simulink model "sampleModel7293_pp_1_1_mu"  (R2018a)
settings: Solver=VariableStepAuto  StartTime=0.0  StopTime=10.0  RelTol=1e-3
undefined symbols (not defined in the file): DiscIntNeverNeededParam
libraries: simulink x367
(part 9 of 13)

== system sampleModel7293_pp_1_1_mu/cfblk193/emi_96 ==
  Action Port : ActionPort  ActionType=else
  emi_97 : Assertion

== system sampleModel7293_pp_1_1_mu/cfblk194/cfblk4 ==
  emi_516 : Inport
  Action Port : ActionPort  ActionType=then
  cfblk4 : simulink/Continuous/PID Controller  Controller=PID  TimeDomain=Discrete-time  SampleTime=-1  IntegratorMethod=Forward Euler  FilterMethod=Forward Euler  Form=Parallel  UseFilter=on  ControllerParametersSource=internal  P=1  I=1  D=0  N=100  InitialConditionSource=internal  InitialConditionForIntegrator=0  InitialConditionForFilter=0  ExternalReset=none  LimitOutput=off  UpperSaturationLimit=inf  LowerSaturationLimit=-inf  LinearizeAsGain=off  AntiWindupMode=none  Kb=1  TrackingMode=off  Kt=1  PParamMin=[]  PParamMax=[]  IParamMin=[]  IParamMax=[]  DParamMin=[]  DParamMax=[]  NParamMin=[]  NParamMax=[]  KbParamMin=[]  KbParamMax=[]  KtParamMin=[]  KtParamMax=[]  POutMin=[]  POutMax=[]  IOutMin=[]  IOutMax=[]  DOutMin=[]  DOutMax=[]  NOutMin=[]  NOutMax=[]  KbOutMin=[]  KbOutMax=[]  KtOutMin=[]  KtOutMax=[]  IntegratorOutMin=[]  IntegratorOutMax=[]  FilterOutMin=[]  FilterOutMax=[]  SumOutMin=[]  SumOutMax=[]  SumI1OutMin=[]  SumI1OutMax=[]  SumI2OutMin=[]  SumI2OutMax=[]  SumI3OutMin=[]  SumI3OutMax=[]  SumDOutMin=[]  SumDOutMax=[]  SaturationOutMin=[]  SaturationOutMax=[]  IntegratorContinuousStateAttributes=''  IntegratorStateMustResolveToSignalObject=off  IntegratorRTWStateStorageClass=Auto  FilterContinuousStateAttributes=''  FilterStateMustResolveToSignalObject=off  FilterRTWStateStorageClass=Auto  DifferentiatorICPrevScaledInput=0  DifferentiatorOutMin=[]  DifferentiatorOutMax=[]  FilterDiffOutCoefMin=[]  FilterDiffOutCoefMax=[]  SumDenOutMin=[]  SumDenOutMax=[]  SumNumOutMin=[]  SumNumOutMax=[]  ReciprocalOutMin=[]  ReciprocalOutMax=[]  DivideOutMin=[]  DivideOutMax=[]  TunerSelectOption=Transfer Function Based (PID Tuner App)
  emi_517 : Outport
  wires:
  emi_516/1 -> cfblk4/1
  cfblk4/1 -> emi_517/1

== system sampleModel7293_pp_1_1_mu/cfblk194/cfblk5 ==
  emi_509 : Inport
  Action Port : ActionPort  ActionType=then
  cfblk5 : UnitDelay  SampleTime=-1
  emi_510 : Outport
  wires:
  emi_509/1 -> cfblk5/1
  cfblk5/1 -> emi_510/1

== system sampleModel7293_pp_1_1_mu/cfblk194/cfblk6 ==
  emi_208 : Inport
  Action Port : ActionPort  ActionType=then
  cfblk6 : DiscreteTransferFcn
  emi_209 : Outport
  wires:
  emi_208/1 -> cfblk6/1
  cfblk6/1 -> emi_209/1

== system sampleModel7293_pp_1_1_mu/cfblk194/cfblk7 ==
  emi_64 : Inport
  emi_65 : Inport  Port=2
  Action Port : ActionPort  ActionType=then
  cfblk7 : Delay  ShowEnablePort=on
      settings: InputPortMap=u0,e6
  emi_66 : Outport
  wires:
  emi_64/1 -> cfblk7/1
  emi_65/1 -> cfblk7/2
  cfblk7/1 -> emi_66/1

== system sampleModel7293_pp_1_1_mu/cfblk194/cfblk8 ==
  emi_1728 : Inport
  Action Port : ActionPort  ActionType=then
  cfblk8 : Delay
  emi_1729 : Outport
  wires:
  emi_1728/1 -> cfblk8/1
  cfblk8/1 -> emi_1729/1

== system sampleModel7293_pp_1_1_mu/cfblk194/emi_1730 ==
  Action Port : ActionPort  ActionType=else
  emi_1731 : Assertion

== system sampleModel7293_pp_1_1_mu/cfblk194/emi_210 ==
  Action Port : ActionPort  ActionType=else
  emi_211 : Assertion

== system sampleModel7293_pp_1_1_mu/cfblk194/emi_511 ==
  Action Port : ActionPort  ActionType=else
  emi_512 : Assertion

== system sampleModel7293_pp_1_1_mu/cfblk194/emi_518 ==
  Action Port : ActionPort  ActionType=else
  emi_519 : Assertion

== system sampleModel7293_pp_1_1_mu/cfblk194/emi_67 ==
  Action Port : ActionPort  ActionType=else
  emi_68 : Assertion

== system sampleModel7293_pp_1_1_mu/cfblk195/cfblk11 ==
  emi_157 : Inport
  Action Port : ActionPort  ActionType=then
  cfblk11 : Delay
  emi_158 : Outport
  wires:
  emi_157/1 -> cfblk11/1
  cfblk11/1 -> emi_158/1

== system sampleModel7293_pp_1_1_mu/cfblk195/cfblk4 ==
  emi_387 : Inport
  Action Port : ActionPort  ActionType=then
  cfblk4 : simulink/Discrete/Difference  ICPrevInput=0.0  OutMin=[]  OutMax=[]  OutDataTypeStr=double  OutputDataTypeScalingMode=double  OutDataType=fixdt(1, 16)  OutScaling=2^-10  DoSatur=off
  emi_388 : Outport
  wires:
  emi_387/1 -> cfblk4/1
  cfblk4/1 -> emi_388/1

== system sampleModel7293_pp_1_1_mu/cfblk195/cfblk8 ==
  cfblk1 : Inport
  cfblk11 : Inport  Port=2
  cfblk12 : Inport  Port=3
  Action Port : ActionPort  ActionType=then
  cfblk10 : simulink/Continuous/PID Controller (2DOF)  Controller=PID  TimeDomain=Discrete-time  SampleTime=-1  IntegratorMethod=Forward Euler  FilterMethod=Forward Euler  Form=Parallel  UseFilter=on  ControllerParametersSource=internal  P=1  I=1  D=0  N=100  b=1  c=1  InitialConditionSource=internal  InitialConditionForIntegrator=0  InitialConditionForFilter=0  ExternalReset=none  LimitOutput=off  UpperSaturationLimit=inf  LowerSaturationLimit=-inf  LinearizeAsGain=off  AntiWindupMode=none  Kb=1  TrackingMode=off  Kt=1  PParamMin=[]  PParamMax=[]  IParamMin=[]  IParamMax=[]  DParamMin=[]  DParamMax=[]  NParamMin=[]  NParamMax=[]  bParamMin=[]  bParamMax=[]  cParamMin=[]  cParamMax=[]  KbParamMin=[]  KbParamMax=[]  KtParamMin=[]  KtParamMax=[]  POutMin=[]  POutMax=[]  IOutMin=[]  IOutMax=[]  DOutMin=[]  DOutMax=[]  NOutMin=[]  NOutMax=[]  bOutMin=[]  bOutMax=[]  cOutMin=[]  cOutMax=[]  KbOutMin=[]  KbOutMax=[]  KtOutMin=[]  KtOutMax=[]  IntegratorOutMin=[]  IntegratorOutMax=[]  FilterOutMin=[]  FilterOutMax=[]  SumOutMin=[]  SumOutMax=[]  Sum1OutMin=[]  Sum1OutMax=[]  Sum2OutMin=[]  Sum2OutMax=[]  Sum3OutMin=[]  Sum3OutMax=[]  SumI1OutMin=[]  SumI1OutMax=[]  SumI2OutMin=[]  SumI2OutMax=[]  SumI3OutMin=[]  SumI3OutMax=[]  SumDOutMin=[]  SumDOutMax=[]  SaturationOutMin=[]  SaturationOutMax=[]  IntegratorContinuousStateAttributes=''  IntegratorStateMustResolveToSignalObject=off  IntegratorRTWStateStorageClass=Auto  FilterContinuousStateAttributes=''  FilterStateMustResolveToSignalObject=off  FilterRTWStateStorageClass=Auto  DifferentiatorICPrevScaledInput=0  DifferentiatorOutMin=[]  DifferentiatorOutMax=[]  FilterDiffOutCoefMin=[]  FilterDiffOutCoefMax=[]  SumDenOutMin=[]  SumDenOutMax=[]  SumNumOutMin=[]  SumNumOutMax=[]  ReciprocalOutMin=[]  ReciprocalOutMax=[]  DivideOutMin=[]  DivideOutMax=[]  TunerSelectOption=Transfer Function Based (PID Tuner App)
  cfblk13 : Subsystem  TreatAsAtomicUnit=on
  cfblk3 : simulink/Discrete/Transfer Fcn Real Zero  ZeroZ=0.75  ICPrevInput=0.0  DoSatur=off
      settings: SourceProductName=Simulink  SourceProductBaseCode=SL
  cfblk4 : Delay  ShowEnablePort=on
      settings: InputPortMap=u0,e6
  cfblk5 : simulink/Discrete/Transfer Fcn First Order  PoleZ=0.95  ICPrevOutput=0.0  DoSatur=off
      settings: SourceProductName=Simulink
  cfblk6 : UnitDelay  SampleTime=-1
  cfblk7 : UnitDelay  SampleTime=-1
  cfblk8 : Subsystem  TreatAsAtomicUnit=on
  cfblk9 : Subsystem  TreatAsAtomicUnit=on
  cyemi_{892..902} (11 alike) : DataTypeConversion  OutDataTypeStr=double
  emi_1595 : Subsystem  TreatAsAtomicUnit=on
  emi_1597 : If  IfExpression=Inf <= u1
  emi_1598 : DataTypeConversion  OutDataTypeStr=double
  emi_1993 : Subsystem  TreatAsAtomicUnit=on
  emi_1995 : If  IfExpression=Inf <= u1
  emi_1996 : DataTypeConversion  OutDataTypeStr=double
  emi_497 : Subsystem  TreatAsAtomicUnit=on
  emi_499 : If  IfExpression=Inf <= u1
  emi_500 : DataTypeConversion  OutDataTypeStr=double
  cfblk2 : Outport
  wires:
  cfblk4/1 -> cyemi_898/1, cyemi_899/1
  cfblk10/1 -> cfblk2/1
  cyemi_892/1 -> cfblk10/1
  cfblk7/1 -> cyemi_892/1, emi_1598/1, emi_1996/1
  cyemi_893/1 -> cfblk10/2
  cfblk3/1 -> cyemi_893/1
  cyemi_895/1 -> cfblk3/1
  cfblk1/1 -> cyemi_895/1
  cyemi_896/1 -> cfblk4/1
  cfblk11/1 -> cyemi_896/1
  cyemi_897/1 -> cfblk4/2
  cyemi_898/1 -> cfblk5/1
  cyemi_899/1 -> cfblk6/1
  cyemi_900/1 -> cfblk7/1
  cfblk12/1 -> cyemi_900/1
  cfblk6/1 -> cyemi_902/1
  cyemi_901/1 -> cfblk8/1(emi_495)
  cfblk8/1(emi_496) -> cyemi_894/1
  emi_499/1 -> cfblk8/Action
  emi_499/2 -> emi_497/Action
  emi_500/1 -> emi_499/1
  cyemi_894/1 -> cfblk13/1(emi_1593)
  cfblk13/1(emi_1594) -> emi_500/1, cyemi_897/1
  emi_1597/1 -> cfblk13/Action
  emi_1597/2 -> emi_1595/Action
  emi_1598/1 -> emi_1597/1
  cyemi_902/1 -> cfblk9/1(emi_1991)
  cfblk9/1(emi_1992) -> cyemi_901/1
  emi_1995/1 -> cfblk9/Action
  emi_1995/2 -> emi_1993/Action
  emi_1996/1 -> emi_1995/1

== system sampleModel7293_pp_1_1_mu/cfblk195/cfblk9 ==
  cfblk1 : Inport
  cfblk11 : Inport  Port=2
  cfblk12 : Inport  Port=3
  cfblk13 : Inport  Port=4
  Action Port : ActionPort  ActionType=else
  cfblk10 : DiscreteZeroPole  Poles=[0 0.5]  Gain=1  SampleTime=-1
  cfblk3 : simulink/Discrete/Transfer Fcn Real Zero  ZeroZ=0.75  ICPrevInput=0.0  DoSatur=off
      settings: SourceProductName=Simulink  SourceProductBaseCode=SL
  cfblk4 : DiscreteFir
  cfblk5 : DiscreteFilter
  cfblk6 : Delay  ShowEnablePort=on
      settings: InputPortMap=u0,e6
  cfblk7 : DiscreteIntegrator  SampleTime=-1  OutDataTypeStr=double  ICPrevOutput=DiscIntNeverNeededParam  ICPrevScaledInput=DiscIntNeverNeededParam
  cfblk8 : UnitDelay  SampleTime=-1
  cfblk9 : Subsystem  TreatAsAtomicUnit=on
  cyemi_{907..915} (9 alike) : DataTypeConversion  OutDataTypeStr=double
  emi_1588 : Subsystem  TreatAsAtomicUnit=on
  emi_1590 : If  IfExpression=0 <= u1
  emi_1591 : DataTypeConversion  OutDataTypeStr=double
  cfblk2 : Outport
  cfblk14 : Outport  Port=2
  cfblk15 : Outport  Port=3
  wires:
  cfblk12/1 -> cfblk2/1
  cfblk6/1 -> cfblk14/1
  cyemi_907/1 -> cfblk10/1
  cfblk13/1 -> cyemi_907/1
  cyemi_908/1 -> cfblk3/1
  cfblk11/1 -> cyemi_908/1
  cyemi_909/1 -> cfblk4/1
  cfblk8/1 -> cyemi_909/1
  cyemi_910/1 -> cfblk5/1
  cfblk4/1 -> cyemi_910/1, emi_1591/1
  cyemi_911/1 -> cfblk6/1
  cfblk5/1 -> cyemi_911/1
  cyemi_912/1 -> cfblk6/2
  cfblk7/1 -> cyemi_912/1
  cyemi_913/1 -> cfblk7/1
  cfblk10/1 -> cyemi_913/1
  cyemi_914/1 -> cfblk8/1
  cfblk3/1 -> cyemi_914/1
  cfblk1/1 -> cyemi_915/1
  cyemi_915/1 -> cfblk9/1(emi_1586)
  cfblk9/1(emi_1587) -> cfblk15/1
  emi_1590/1 -> cfblk9/Action
  emi_1590/2 -> emi_1588/Action
  emi_1591/1 -> emi_1590/1

== system sampleModel7293_pp_1_1_mu/cfblk195/emi_159 ==
  Action Port : ActionPort  ActionType=else
  emi_160 : Assertion

== system sampleModel7293_pp_1_1_mu/cfblk195/emi_389 ==
  Action Port : ActionPort  ActionType=else
  emi_390 : Assertion

== system sampleModel7293_pp_1_1_mu/cfblk196/cfblk11 ==
  cfblk1 : Inport
  cfblk10 : Inport  Port=2
  cfblk11 : Inport  Port=3
  Action Port : ActionPort  ActionType=then
  cfblk3 : Subsystem  TreatAsAtomicUnit=on
  cfblk4 : DiscreteStateSpace  SampleTime=-1
  cfblk5 : simulink/Discrete/Transfer Fcn First Order  PoleZ=0.95  ICPrevOutput=0.0  DoSatur=off
      settings: SourceProductName=Simulink
  cfblk6 : simulink/Discrete/Transfer Fcn First Order  PoleZ=0.95  ICPrevOutput=0.0  DoSatur=off
      settings: SourceProductName=Simulink
  cfblk7 : DiscreteFilter
  cfblk8 : simulink/Discrete/Transfer Fcn Lead or Lag  PoleZ=0.95  ZeroZ=0.75  ICPrevOutput=0.0  ICPrevInput=0.0  DoSatur=off
      settings: SourceProductName=Simulink  SourceProductBaseCode=SL
  cfblk9 : simulink/Discrete/Tapped Delay  vinit=0.0  samptime=-1  NumDelays=1  DelayOrder=Oldest  includeCurrent=off
  cyemi_{922..928} (7 alike) : DataTypeConversion  OutDataTypeStr=double
  emi_1152 : Subsystem  TreatAsAtomicUnit=on
  emi_1154 : If  IfExpression=Inf <= u1
  emi_1155 : DataTypeConversion  OutDataTypeStr=double
  cfblk2 : Outport
  cfblk12 : Outport  Port=2
  cfblk13 : Outport  Port=3
  wires:
  cfblk4/1 -> cfblk13/1, emi_1155/1
  cfblk9/1 -> cfblk2/1
  cfblk1/1 -> cyemi_924/1, cyemi_925/1
  cfblk7/1 -> cyemi_922/1
  cyemi_923/1 -> cfblk4/1
  cfblk6/1 -> cyemi_923/1
  cyemi_924/1 -> cfblk5/1
  cyemi_925/1 -> cfblk6/1
  cyemi_926/1 -> cfblk7/1
  cfblk8/1 -> cyemi_926/1
  cyemi_927/1 -> cfblk8/1
  cfblk11/1 -> cyemi_927/1
  cyemi_928/1 -> cfblk9/1
  cfblk10/1 -> cyemi_928/1
  cyemi_922/1 -> cfblk3/1(emi_1150)
  cfblk3/1(emi_1151) -> cfblk12/1
  emi_1154/1 -> cfblk3/Action
  emi_1154/2 -> emi_1152/Action
  emi_1155/1 -> emi_1154/1

== system sampleModel7293_pp_1_1_mu/cfblk196/cfblk12 ==
  cfblk1 : Inport
  Action Port : ActionPort  ActionType=else
  cfblk10 : DiscreteZeroPole  Poles=[0 0.5]  Gain=1  SampleTime=-1
  cfblk11 : DiscreteIntegrator  SampleTime=-1  OutDataTypeStr=double  ICPrevOutput=DiscIntNeverNeededParam  ICPrevScaledInput=DiscIntNeverNeededParam
  cfblk13 : Delay
  cfblk3 : Subsystem  TreatAsAtomicUnit=on
  cfblk4 : DiscreteFir
  cfblk5 : simulink/Discrete/Transfer Fcn Lead or Lag  PoleZ=0.95  ZeroZ=0.75  ICPrevOutput=0.0  ICPrevInput=0.0  DoSatur=off
      settings: SourceProductName=Simulink  SourceProductBaseCode=SL
  cfblk6 : DiscreteFir
  cfblk7 : simulink/Discrete/Difference  ICPrevInput=0.0  OutMin=[]  OutMax=[]  OutDataTypeStr=double  OutputDataTypeScalingMode=double  OutDataType=fixdt(1, 16)  OutScaling=2^-10  DoSatur=off
  cfblk8 : DiscreteFilter
  cfblk9 : Subsystem  TreatAsAtomicUnit=on
  cyemi_{930..939} (10 alike) : DataTypeConversion  OutDataTypeStr=double
  emi_1823 : Subsystem  TreatAsAtomicUnit=on
  emi_1825 : If  IfExpression=Inf <= u1
  emi_1826 : DataTypeConversion  OutDataTypeStr=double
  emi_569 : Subsystem  TreatAsAtomicUnit=on
  emi_571 : If  IfExpression=Inf <= u1
  emi_572 : DataTypeConversion  OutDataTypeStr=double
  cfblk2 : Outport
  cfblk12 : Outport  Port=2
  wires:
  cfblk10/1 -> cfblk12/1, cfblk2/1
  cyemi_930/1 -> cfblk10/1
  cfblk5/1 -> cyemi_930/1
  cyemi_931/1 -> cfblk11/1
  cfblk8/1 -> cyemi_931/1
  cyemi_932/1 -> cfblk13/1
  cfblk4/1 -> cyemi_933/1, emi_572/1, emi_1826/1
  cyemi_934/1 -> cfblk4/1
  cfblk11/1 -> cyemi_934/1
  cyemi_935/1 -> cfblk5/1
  cyemi_936/1 -> cfblk6/1
  cfblk13/1 -> cyemi_936/1
  cyemi_937/1 -> cfblk7/1
  cfblk1/1 -> cyemi_937/1
  cyemi_938/1 -> cfblk8/1
  cfblk7/1 -> cyemi_938/1
  cfblk6/1 -> cyemi_939/1
  cyemi_939/1 -> cfblk9/1(emi_567)
  cfblk9/1(emi_568) -> cyemi_932/1
  emi_571/1 -> cfblk9/Action
  emi_571/2 -> emi_569/Action
  emi_572/1 -> emi_571/1
  cyemi_933/1 -> cfblk3/1(emi_1821)
  cfblk3/1(emi_1822) -> cyemi_935/1
  emi_1825/1 -> cfblk3/Action
  emi_1825/2 -> emi_1823/Action
  emi_1826/1 -> emi_1825/1

== system sampleModel7293_pp_1_1_mu/cfblk196/cfblk3 ==
  emi_229 : Inport
  Action Port : ActionPort  ActionType=then
  cfblk3 : simulink/Continuous/PID Controller  Controller=PID  TimeDomain=Discrete-time  SampleTime=-1  IntegratorMethod=Forward Euler  FilterMethod=Forward Euler  Form=Parallel  UseFilter=on  ControllerParametersSource=internal  P=1  I=1  D=0  N=100  InitialConditionSource=internal  InitialConditionForIntegrator=0  InitialConditionForFilter=0  ExternalReset=none  LimitOutput=off  UpperSaturationLimit=inf  LowerSaturationLimit=-inf  LinearizeAsGain=off  AntiWindupMode=none  Kb=1  TrackingMode=off  Kt=1  PParamMin=[]  PParamMax=[]  IParamMin=[]  IParamMax=[]  DParamMin=[]  DParamMax=[]  NParamMin=[]  NParamMax=[]  KbParamMin=[]  KbParamMax=[]  KtParamMin=[]  KtParamMax=[]  POutMin=[]  POutMax=[]  IOutMin=[]  IOutMax=[]  DOutMin=[]  DOutMax=[]  NOutMin=[]  NOutMax=[]  KbOutMin=[]  KbOutMax=[]  KtOutMin=[]  KtOutMax=[]  IntegratorOutMin=[]  IntegratorOutMax=[]  FilterOutMin=[]  FilterOutMax=[]  SumOutMin=[]  SumOutMax=[]  SumI1OutMin=[]  SumI1OutMax=[]  SumI2OutMin=[]  SumI2OutMax=[]  SumI3OutMin=[]  SumI3OutMax=[]  SumDOutMin=[]  SumDOutMax=[]  SaturationOutMin=[]  SaturationOutMax=[]  IntegratorContinuousStateAttributes=''  IntegratorStateMustResolveToSignalObject=off  IntegratorRTWStateStorageClass=Auto  FilterContinuousStateAttributes=''  FilterStateMustResolveToSignalObject=off  FilterRTWStateStorageClass=Auto  DifferentiatorICPrevScaledInput=0  DifferentiatorOutMin=[]  DifferentiatorOutMax=[]  FilterDiffOutCoefMin=[]  FilterDiffOutCoefMax=[]  SumDenOutMin=[]  SumDenOutMax=[]  SumNumOutMin=[]  SumNumOutMax=[]  ReciprocalOutMin=[]  ReciprocalOutMax=[]  DivideOutMin=[]  DivideOutMax=[]  TunerSelectOption=Transfer Function Based (PID Tuner App)
  emi_230 : Outport
  wires:
  emi_229/1 -> cfblk3/1
  cfblk3/1 -> emi_230/1

== system sampleModel7293_pp_1_1_mu/cfblk196/cfblk4 ==
  emi_308 : Inport
  Action Port : ActionPort  ActionType=then
  cfblk4 : simulink/Discrete/Transfer Fcn Lead or Lag  PoleZ=0.95  ZeroZ=0.75  ICPrevOutput=0.0  ICPrevInput=0.0  DoSatur=off
      settings: SourceProductName=Simulink  SourceProductBaseCode=SL
  emi_309 : Outport
  wires:
  emi_308/1 -> cfblk4/1
  cfblk4/1 -> emi_309/1

== system sampleModel7293_pp_1_1_mu/cfblk196/cfblk7 ==
  emi_1657 : Inport
  Action Port : ActionPort  ActionType=then
  cfblk7 : DiscreteIntegrator  SampleTime=-1  OutDataTypeStr=double  ICPrevOutput=DiscIntNeverNeededParam  ICPrevScaledInput=DiscIntNeverNeededParam
  emi_1658 : Outport
  wires:
  emi_1657/1 -> cfblk7/1
  cfblk7/1 -> emi_1658/1

== system sampleModel7293_pp_1_1_mu/cfblk196/emi_1659 ==
  Action Port : ActionPort  ActionType=else
  emi_1660 : Assertion

== system sampleModel7293_pp_1_1_mu/cfblk196/emi_231 ==
  Action Port : ActionPort  ActionType=else
  emi_232 : Assertion

== system sampleModel7293_pp_1_1_mu/cfblk196/emi_310 ==
  Action Port : ActionPort  ActionType=else
  emi_311 : Assertion

== system sampleModel7293_pp_1_1_mu/cfblk197/cfblk16 ==
  cfblk1 : Inport
  Action Port : ActionPort  ActionType=then
  cfblk10 : DiscreteIntegrator  SampleTime=-1  OutDataTypeStr=double  ICPrevOutput=DiscIntNeverNeededParam  ICPrevScaledInput=DiscIntNeverNeededParam
  cfblk{8,14..16} (4 alike) : Delay
  cfblk3 : simulink/Discrete/Difference  ICPrevInput=0.0  OutMin=[]  OutMax=[]  OutDataTypeStr=double  OutputDataTypeScalingMode=double  OutDataType=fixdt(1, 16)  OutScaling=2^-10  DoSatur=off
  cfblk4 : Subsystem  TreatAsAtomicUnit=on
  cfblk5 : simulink/Continuous/PID Controller (2DOF)  Controller=PID  TimeDomain=Discrete-time  SampleTime=-1  IntegratorMethod=Forward Euler  FilterMethod=Forward Euler  Form=Parallel  UseFilter=on  ControllerParametersSource=internal  P=1  I=1  D=0  N=100  b=1  c=1  InitialConditionSource=internal  InitialConditionForIntegrator=0  InitialConditionForFilter=0  ExternalReset=none  LimitOutput=off  UpperSaturationLimit=inf  LowerSaturationLimit=-inf  LinearizeAsGain=off  AntiWindupMode=none  Kb=1  TrackingMode=off  Kt=1  PParamMin=[]  PParamMax=[]  IParamMin=[]  IParamMax=[]  DParamMin=[]  DParamMax=[]  NParamMin=[]  NParamMax=[]  bParamMin=[]  bParamMax=[]  cParamMin=[]  cParamMax=[]  KbParamMin=[]  KbParamMax=[]  KtParamMin=[]  KtParamMax=[]  POutMin=[]  POutMax=[]  IOutMin=[]  IOutMax=[]  DOutMin=[]  DOutMax=[]  NOutMin=[]  NOutMax=[]  bOutMin=[]  bOutMax=[]  cOutMin=[]  cOutMax=[]  KbOutMin=[]  KbOutMax=[]  KtOutMin=[]  KtOutMax=[]  IntegratorOutMin=[]  IntegratorOutMax=[]  FilterOutMin=[]  FilterOutMax=[]  SumOutMin=[]  SumOutMax=[]  Sum1OutMin=[]  Sum1OutMax=[]  Sum2OutMin=[]  Sum2OutMax=[]  Sum3OutMin=[]  Sum3OutMax=[]  SumI1OutMin=[]  SumI1OutMax=[]  SumI2OutMin=[]  SumI2OutMax=[]  SumI3OutMin=[]  SumI3OutMax=[]  SumDOutMin=[]  SumDOutMax=[]  SaturationOutMin=[]  SaturationOutMax=[]  IntegratorContinuousStateAttributes=''  IntegratorStateMustResolveToSignalObject=off  IntegratorRTWStateStorageClass=Auto  FilterContinuousStateAttributes=''  FilterStateMustResolveToSignalObject=off  FilterRTWStateStorageClass=Auto  DifferentiatorICPrevScaledInput=0  DifferentiatorOutMin=[]  DifferentiatorOutMax=[]  FilterDiffOutCoefMin=[]  FilterDiffOutCoefMax=[]  SumDenOutMin=[]  SumDenOutMax=[]  SumNumOutMin=[]  SumNumOutMax=[]  ReciprocalOutMin=[]  ReciprocalOutMax=[]  DivideOutMin=[]  DivideOutMax=[]  TunerSelectOption=Transfer Function Based (PID Tuner App)
  cfblk6 : UnitDelay  SampleTime=-1
  cfblk7 : simulink/Discrete/Transfer Fcn First Order  PoleZ=0.95  ICPrevOutput=0.0  DoSatur=off
      settings: SourceProductName=Simulink
  cfblk9 : Subsystem  TreatAsAtomicUnit=on
  cyemi_{956..967} (12 alike) : DataTypeConversion  OutDataTypeStr=double
  emi_1452 : Subsystem  TreatAsAtomicUnit=on
  emi_1454 : If  IfExpression=Inf <= u1
  emi_1455 : DataTypeConversion  OutDataTypeStr=double
  emi_1887 : Subsystem  TreatAsAtomicUnit=on
  emi_1889 : If  IfExpression=Inf <= u1
  emi_1890 : DataTypeConversion  OutDataTypeStr=double
  cfblk2 : Outport
  cfblk11 : Outport  Port=2
  cfblk12 : Outport  Port=3
  cfblk13 : Outport  Port=4
  wires:
  cfblk10/1 -> cyemi_958/1, cyemi_959/1, emi_1890/1
  cfblk5/1 -> cfblk11/1, cfblk2/1, cyemi_956/1
  cfblk1/1 -> cfblk13/1
  cfblk7/1 -> cfblk12/1, cyemi_967/1
  cyemi_956/1 -> cfblk10/1
  cyemi_957/1 -> cfblk14/1
  cfblk8/1 -> cyemi_957/1
  cyemi_958/1 -> cfblk15/1
  cyemi_959/1 -> cfblk16/1
  cyemi_960/1 -> cfblk3/1
  cfblk14/1 -> cyemi_960/1
  cfblk3/1 -> cyemi_961/1
  cyemi_962/1 -> cfblk5/1
  cfblk15/1 -> cyemi_962/1, emi_1455/1
  cyemi_963/1 -> cfblk5/2
  cfblk16/1 -> cyemi_963/1
  cyemi_964/1 -> cfblk6/1
  cyemi_965/1 -> cfblk7/1
  cyemi_966/1 -> cfblk8/1
  cfblk6/1 -> cyemi_966/1
  cyemi_967/1 -> cfblk9/1(emi_1450)
  cfblk9/1(emi_1451) -> cyemi_964/1
  emi_1454/1 -> cfblk9/Action
  emi_1454/2 -> emi_1452/Action
  emi_1455/1 -> emi_1454/1
  cyemi_961/1 -> cfblk4/1(emi_1885)
  cfblk4/1(emi_1886) -> cyemi_965/1
  emi_1889/1 -> cfblk4/Action
  emi_1889/2 -> emi_1887/Action
  emi_1890/1 -> emi_1889/1

== system sampleModel7293_pp_1_1_mu/cfblk197/cfblk17 ==
  cfblk1 : Inport
  cfblk12 : Inport  Port=2
  cfblk13 : Inport  Port=3
  cfblk14 : Inport  Port=4
  Action Port : ActionPort  ActionType=else
  cfblk10 : DiscreteIntegrator  SampleTime=-1  OutDataTypeStr=double  ICPrevOutput=DiscIntNeverNeededParam  ICPrevScaledInput=DiscIntNeverNeededParam
  cfblk11 : DiscreteIntegrator  SampleTime=-1  OutDataTypeStr=double  ICPrevOutput=DiscIntNeverNeededParam  ICPrevScaledInput=DiscIntNeverNeededParam
  cfblk16 : Subsystem  TreatAsAtomicUnit=on
  cfblk3 : simulink/Discrete/Transfer Fcn First Order  PoleZ=0.95  ICPrevOutput=0.0  DoSatur=off
      settings: SourceProductName=Simulink
  cfblk4 : Subsystem  TreatAsAtomicUnit=on
  cfblk5 : Delay  ShowEnablePort=on
      settings: InputPortMap=u0,e6
  cfblk6 : Subsystem  TreatAsAtomicUnit=on
  cfblk7 : Delay  DelayLengthSource=Input port
      settings: InputPortMap=u0,p1
  cfblk8 : simulink/Discrete/Tapped Delay  vinit=0.0  samptime=-1  NumDelays=1  DelayOrder=Oldest  includeCurrent=off
  cfblk9 : Delay  DelayLengthSource=Input port
      settings: InputPortMap=u0,p1
  cyemi_{972..981,983} (11 alike) : DataTypeConversion  OutDataTypeStr=double
  cyemi_982 : DataTypeConversion  OutDataTypeStr=uint32
  cyemi_984 : DataTypeConversion  OutDataTypeStr=uint32
  emi_1325 : Subsystem  TreatAsAtomicUnit=on
  emi_1327 : If  IfExpression=0 <= u1
  emi_1328 : DataTypeConversion  OutDataTypeStr=double
  emi_1781 : Subsystem  TreatAsAtomicUnit=on
  emi_1783 : If  IfExpression=0 <= u1
  emi_1784 : DataTypeConversion  OutDataTypeStr=double
  emi_769 : Subsystem  TreatAsAtomicUnit=on
  emi_771 : If  IfExpression=0 <= u1
  emi_772 : DataTypeConversion  OutDataTypeStr=double
  cfblk2 : Outport
  cfblk15 : Outport  Port=2
  wires:
  cfblk1/1 -> cfblk15/1
  cfblk3/1 -> cyemi_981/1, cyemi_983/1
  cyemi_972/1 -> cfblk10/1
  cyemi_973/1 -> cfblk11/1
  cfblk13/1 -> cyemi_973/1
  cfblk7/1 -> cyemi_974/1
  cyemi_975/1 -> cfblk3/1
  cfblk5/1 -> cyemi_976/1, emi_1328/1
  cyemi_977/1 -> cfblk5/1
  cfblk9/1 -> cyemi_977/1, emi_772/1
  cyemi_978/1 -> cfblk5/2
  cfblk10/1 -> cyemi_978/1
  cfblk11/1 -> cyemi_979/1, emi_1784/1
  cyemi_980/1 -> cfblk7/1
  cfblk14/1 -> cyemi_980/1
  cyemi_981/1 -> cfblk7/2
  cyemi_982/1 -> cfblk8/1
  cfblk12/1 -> cyemi_982/1
  cyemi_983/1 -> cfblk9/1
  cyemi_984/1 -> cfblk9/2
  cfblk8/1 -> cyemi_984/1
  cyemi_979/1 -> cfblk6/1(emi_767)
  cfblk6/1(emi_768) -> cyemi_972/1
  emi_771/1 -> cfblk6/Action
  emi_771/2 -> emi_769/Action
  emi_772/1 -> emi_771/1
  cyemi_976/1 -> cfblk4/1(emi_1323)
  cfblk4/1(emi_1324) -> cfblk2/1
  emi_1327/1 -> cfblk4/Action
  emi_1327/2 -> emi_1325/Action
  emi_1328/1 -> emi_1327/1
  cyemi_974/1 -> cfblk16/1(emi_1779)
  cfblk16/1(emi_1780) -> cyemi_975/1
  emi_1783/1 -> cfblk16/Action
  emi_1783/2 -> emi_1781/Action
  emi_1784/1 -> emi_1783/1

== system sampleModel7293_pp_1_1_mu/cfblk197/cfblk18 ==
  emi_1078 : Inport
  Action Port : ActionPort  ActionType=then
  cfblk18 : Delay
  emi_1079 : Outport
  wires:
  emi_1078/1 -> cfblk18/1
  cfblk18/1 -> emi_1079/1

== system sampleModel7293_pp_1_1_mu/cfblk197/cfblk19 ==
  emi_429 : Inport
  Action Port : ActionPort  ActionType=then
  cfblk19 : Delay
  emi_430 : Outport
  wires:
  emi_429/1 -> cfblk19/1
  cfblk19/1 -> emi_430/1

== system sampleModel7293_pp_1_1_mu/cfblk197/cfblk25 ==
  emi_1955 : Inport
  Action Port : ActionPort  ActionType=then
  cfblk25 : DataTypeConversion  OutDataTypeStr=double
  emi_1956 : Outport
  wires:
  emi_1955/1 -> cfblk25/1
  cfblk25/1 -> emi_1956/1

== system sampleModel7293_pp_1_1_mu/cfblk197/cfblk5 ==
  emi_1365 : Inport
  Action Port : ActionPort  ActionType=then
  cfblk5 : DiscreteTransferFcn
  emi_1366 : Outport
  wires:
  emi_1365/1 -> cfblk5/1
  cfblk5/1 -> emi_1366/1

== system sampleModel7293_pp_1_1_mu/cfblk197/cfblk8 ==
  emi_243 : Inport
  Action Port : ActionPort  ActionType=then
  cfblk8 : DiscreteStateSpace  SampleTime=-1
  emi_244 : Outport
  wires:
  emi_243/1 -> cfblk8/1
  cfblk8/1 -> emi_244/1

== system sampleModel7293_pp_1_1_mu/cfblk197/emi_1080 ==
  Action Port : ActionPort  ActionType=else
  emi_1081 : Assertion

== system sampleModel7293_pp_1_1_mu/cfblk197/emi_1367 ==
  Action Port : ActionPort  ActionType=else
  emi_1368 : Assertion

== system sampleModel7293_pp_1_1_mu/cfblk197/emi_1957 ==
  Action Port : ActionPort  ActionType=else
  emi_1958 : Assertion

== system sampleModel7293_pp_1_1_mu/cfblk197/emi_245 ==
  Action Port : ActionPort  ActionType=else
  emi_246 : Assertion

== system sampleModel7293_pp_1_1_mu/cfblk197/emi_431 ==
  Action Port : ActionPort  ActionType=else
  emi_432 : Assertion

== system sampleModel7293_pp_1_1_mu/cfblk198/cfblk14 ==
  cfblk1 : Inport
  cfblk10 : Inport  Port=2
  Action Port : ActionPort  ActionType=then
  cfblk3 : DiscreteFilter
  cfblk4 : simulink/Discrete/Transfer Fcn First Order  PoleZ=0.95  ICPrevOutput=0.0  DoSatur=off
      settings: SourceProductName=Simulink
  cfblk5 : simulink/Discrete/Tapped Delay  vinit=0.0  samptime=-1  NumDelays=1  DelayOrder=Oldest  includeCurrent=off
  cfblk6 : DiscreteIntegrator  SampleTime=-1  OutDataTypeStr=double  ICPrevOutput=DiscIntNeverNeededParam  ICPrevScaledInput=DiscIntNeverNeededParam
  cfblk7 : Subsystem  TreatAsAtomicUnit=on
  cfblk8 : DiscreteZeroPole  Poles=[0 0.5]  Gain=1  SampleTime=-1
  cfblk9 : Subsystem  TreatAsAtomicUnit=on
  cyemi_{1008..1014} (7 alike) : DataTypeConversion  OutDataTypeStr=double
  emi_1431 : Subsystem  TreatAsAtomicUnit=on
  emi_1433 : If  IfExpression=Inf <= u1
  emi_1434 : DataTypeConversion  OutDataTypeStr=double
  emi_1709 : Subsystem  TreatAsAtomicUnit=on
  emi_1711 : If  IfExpression=Inf <= u1
  emi_1712 : DataTypeConversion  OutDataTypeStr=double
  cfblk2 : Outport
  cfblk11 : Outport  Port=2
  wires:
  cfblk5/1 -> cfblk2/1, emi_1434/1
  cyemi_1008/1 -> cfblk3/1
  cfblk10/1 -> cyemi_1008/1
  cyemi_1009/1 -> cfblk4/1
  cfblk1/1 -> cyemi_1009/1
  cyemi_1010/1 -> cfblk5/1
  cfblk4/1 -> cyemi_1010/1
  cyemi_1011/1 -> cfblk6/1
  cfblk8/1 -> cyemi_1011/1
  cfblk6/1 -> cyemi_1012/1
  cyemi_1013/1 -> cfblk8/1
  cfblk3/1 -> cyemi_1014/1
  cyemi_1012/1 -> cfblk7/1(emi_1429)
  cfblk7/1(emi_1430) -> cfblk11/1, emi_1712/1
  emi_1433/1 -> cfblk7/Action
  emi_1433/2 -> emi_1431/Action
  emi_1434/1 -> emi_1433/1
  cyemi_1014/1 -> cfblk9/1(emi_1707)
  cfblk9/1(emi_1708) -> cyemi_1013/1
  emi_1711/1 -> cfblk9/Action
  emi_1711/2 -> emi_1709/Action
  emi_1712/1 -> emi_1711/1

== system sampleModel7293_pp_1_1_mu/cfblk198/cfblk15 ==
  cfblk1 : Inport
  cfblk6 : Inport  Port=2
  Action Port : ActionPort  ActionType=else
  cfblk3 : simulink/Discrete/Transfer Fcn First Order  PoleZ=0.95  ICPrevOutput=0.0  DoSatur=off
      settings: SourceProductName=Simulink
  cfblk4 : Delay  DelayLengthSource=Input port
      settings: InputPortMap=u0,p1
  cfblk5 : Subsystem  TreatAsAtomicUnit=on
  cyemi_{1017..1020} (4 alike) : DataTypeConversion  OutDataTypeStr=double
  emi_2128 : Subsystem  TreatAsAtomicUnit=on
  emi_2130 : If  IfExpression=Inf <= u1
  emi_2131 : DataTypeConversion  OutDataTypeStr=double
  cfblk2 : Outport
  cfblk7 : Outport  Port=2
  wires:
  cfblk6/1 -> cfblk7/1
  cfblk4/1 -> cfblk2/1, emi_2131/1
  cfblk1/1 -> cyemi_1019/1, cyemi_1020/1
  cyemi_1017/1 -> cfblk3/1
  cyemi_1018/1 -> cfblk4/1
  cfblk3/1 -> cyemi_1018/1
  cyemi_1019/1 -> cfblk4/2
  cyemi_1020/1 -> cfblk5/1(emi_2126)
  cfblk5/1(emi_2127) -> cyemi_1017/1
  emi_2130/1 -> cfblk5/Action
  emi_2130/2 -> emi_2128/Action
  emi_2131/1 -> emi_2130/1

== system sampleModel7293_pp_1_1_mu/cfblk198/cfblk16 ==
  cfblk1 : Inport
  cfblk14 : Inport  Port=2
  Action Port : ActionPort  ActionType=then
  cfblk10 : DiscreteTransferFcn
  cfblk11 : Subsystem  TreatAsAtomicUnit=on
  cfblk12 : simulink/Discrete/Transfer Fcn First Order  PoleZ=0.95  ICPrevOutput=0.0  DoSatur=off
      settings: SourceProductName=Simulink
  cfblk13 : Subsystem  TreatAsAtomicUnit=on
  cfblk16 : Subsystem  TreatAsAtomicUnit=on
  cfblk17 : Subsystem  TreatAsAtomicUnit=on
  cfblk3 : simulink/Discrete/Transfer Fcn Real Zero  ZeroZ=0.75  ICPrevInput=0.0  DoSatur=off
      settings: SourceProductName=Simulink  SourceProductBaseCode=SL
  cfblk4 : Subsystem  TreatAsAtomicUnit=on
  cfblk5 : DiscreteZeroPole  Poles=[0 0.5]  Gain=1  SampleTime=-1
  cfblk6 : simulink/Continuous/PID Controller  Controller=PID  TimeDomain=Discrete-time  SampleTime=-1  IntegratorMethod=Forward Euler  FilterMethod=Forward Euler  Form=Parallel  UseFilter=on  ControllerParametersSource=internal  P=1  I=1  D=0  N=100  InitialConditionSource=internal  InitialConditionForIntegrator=0  InitialConditionForFilter=0  ExternalReset=none  LimitOutput=off  UpperSaturationLimit=inf  LowerSaturationLimit=-inf  LinearizeAsGain=off  AntiWindupMode=none  Kb=1  TrackingMode=off  Kt=1  PParamMin=[]  PParamMax=[]  IParamMin=[]  IParamMax=[]  DParamMin=[]  DParamMax=[]  NParamMin=[]  NParamMax=[]  KbParamMin=[]  KbParamMax=[]  KtParamMin=[]  KtParamMax=[]  POutMin=[]  POutMax=[]  IOutMin=[]  IOutMax=[]  DOutMin=[]  DOutMax=[]  NOutMin=[]  NOutMax=[]  KbOutMin=[]  KbOutMax=[]  KtOutMin=[]  KtOutMax=[]  IntegratorOutMin=[]  IntegratorOutMax=[]  FilterOutMin=[]  FilterOutMax=[]  SumOutMin=[]  SumOutMax=[]  SumI1OutMin=[]  SumI1OutMax=[]  SumI2OutMin=[]  SumI2OutMax=[]  SumI3OutMin=[]  SumI3OutMax=[]  SumDOutMin=[]  SumDOutMax=[]  SaturationOutMin=[]  SaturationOutMax=[]  IntegratorContinuousStateAttributes=''  IntegratorStateMustResolveToSignalObject=off  IntegratorRTWStateStorageClass=Auto  FilterContinuousStateAttributes=''  FilterStateMustResolveToSignalObject=off  FilterRTWStateStorageClass=Auto  DifferentiatorICPrevScaledInput=0  DifferentiatorOutMin=[]  DifferentiatorOutMax=[]  FilterDiffOutCoefMin=[]  FilterDiffOutCoefMax=[]  SumDenOutMin=[]  SumDenOutMax=[]  SumNumOutMin=[]  SumNumOutMax=[]  ReciprocalOutMin=[]  ReciprocalOutMax=[]  DivideOutMin=[]  DivideOutMax=[]  TunerSelectOption=Transfer Function Based (PID Tuner App)
  cfblk7 : DiscreteTransferFcn
  cfblk8 : DiscreteFir
  cfblk9 : DiscreteTransferFcn
  cyemi_{1023..1036} (14 alike) : DataTypeConversion  OutDataTypeStr=double
  emi_1017 : Subsystem  TreatAsAtomicUnit=on
  emi_{168,729,1019,1320,1896} (5 alike) : If  IfExpression=Inf <= u1
  emi_{169,730,1020,1321,1897} (5 alike) : DataTypeConversion  OutDataTypeStr=double
  emi_1318 : Subsystem  TreatAsAtomicUnit=on
  emi_166 : Subsystem  TreatAsAtomicUnit=on
  emi_1894 : Subsystem  TreatAsAtomicUnit=on
  emi_727 : Subsystem  TreatAsAtomicUnit=on
  cfblk2 : Outport
  cfblk15 : Outport  Port=2
  wires:
  cfblk10/1 -> cfblk2/1
  cfblk8/1 -> cfblk15/1, cyemi_1028/1, emi_1020/1
  cyemi_1023/1 -> cfblk10/1
  cfblk14/1 -> cyemi_1024/1
  cyemi_1025/1 -> cfblk12/1
  cfblk3/1 -> cyemi_1025/1
  cfblk7/1 -> cyemi_1026/1
  cfblk12/1 -> cyemi_1027/1
  cyemi_1029/1 -> cfblk3/1
  cfblk1/1 -> cyemi_1030/1
  cyemi_1032/1 -> cfblk5/1
  cfblk9/1 -> cyemi_1032/1, emi_1897/1
  cyemi_1033/1 -> cfblk6/1
  cyemi_1034/1 -> cfblk7/1
  cfblk5/1 -> cyemi_1034/1, emi_1321/1
  cyemi_1035/1 -> cfblk8/1
  cfblk6/1 -> cyemi_1035/1
  cyemi_1036/1 -> cfblk9/1
  cyemi_1026/1 -> cfblk13/1(emi_164)
  cfblk13/1(emi_165) -> cyemi_1023/1
  emi_168/1 -> cfblk13/Action
  emi_168/2 -> emi_166/Action
  emi_169/1 -> emi_168/1
  cyemi_1027/1 -> cfblk16/1(emi_725)
  cfblk16/1(emi_726) -> cyemi_1029/1
  emi_729/1 -> cfblk16/Action
  emi_729/2 -> emi_727/Action
  emi_730/1 -> emi_729/1
  cyemi_1028/1 -> cfblk17/1(emi_1015)
  cfblk17/1(emi_1016) -> cyemi_1033/1
  emi_1019/1 -> cfblk17/Action
  emi_1019/2 -> emi_1017/Action
  emi_1020/1 -> emi_1019/1
  cyemi_1030/1 -> cfblk4/1(emi_1315)
  cyemi_1031/1 -> cfblk4/2(emi_1316)
  cfblk4/1(emi_1317) -> cyemi_1036/1
  emi_1320/1 -> cfblk4/Action
  emi_1320/2 -> emi_1318/Action
  emi_1321/1 -> emi_1320/1
  cyemi_1024/1 -> cfblk11/1(emi_1892)
  cfblk11/1(emi_1893) -> emi_730/1, emi_169/1, cyemi_1031/1
  emi_1896/1 -> cfblk11/Action
  emi_1896/2 -> emi_1894/Action
  emi_1897/1 -> emi_1896/1

== system sampleModel7293_pp_1_1_mu/cfblk198/cfblk17 ==
  cfblk1 : Inport
  cfblk10 : Inport  Port=2
  Action Port : ActionPort  ActionType=else
  cfblk3 : Delay
  cfblk4 : DiscreteFilter
  cfblk5 : simulink/Discrete/Transfer Fcn Real Zero  ZeroZ=0.75  ICPrevInput=0.0  DoSatur=off
      settings: SourceProductName=Simulink  SourceProductBaseCode=SL
  cfblk6 : Subsystem  TreatAsAtomicUnit=on
  cfblk7 : DiscreteIntegrator  SampleTime=-1  OutDataTypeStr=double  ICPrevOutput=DiscIntNeverNeededParam  ICPrevScaledInput=DiscIntNeverNeededParam
  cfblk8 : UnitDelay  SampleTime=-1
  cfblk9 : Subsystem  TreatAsAtomicUnit=on
  cyemi_{1039..1045} (7 alike) : DataTypeConversion  OutDataTypeStr=double
  emi_1609 : Subsystem  TreatAsAtomicUnit=on
  emi_1611 : If  IfExpression=Inf <= u1
  emi_1612 : DataTypeConversion  OutDataTypeStr=double
  emi_445 : Subsystem  TreatAsAtomicUnit=on
  emi_447 : If  IfExpression=Inf <= u1
  emi_448 : DataTypeConversion  OutDataTypeStr=double
  cfblk2 : Outport
  wires:
  cfblk5/1 -> cfblk2/1
  cyemi_1039/1 -> cfblk3/1
  cfblk8/1 -> cyemi_1039/1, emi_448/1
  cyemi_1040/1 -> cfblk4/1
  cyemi_1041/1 -> cfblk5/1
  cfblk1/1 -> cyemi_1041/1
  cfblk10/1 -> cyemi_1042/1
  cyemi_1043/1 -> cfblk7/1
  cfblk3/1 -> cyemi_1043/1
  cyemi_1044/1 -> cfblk8/1
  cfblk7/1 -> cyemi_1045/1, emi_1612/1
  cyemi_1045/1 -> cfblk9/1(emi_443)
  cfblk9/1(emi_444) -> cyemi_1040/1
  emi_447/1 -> cfblk9/Action
  emi_447/2 -> emi_445/Action
  emi_448/1 -> emi_447/1
  cyemi_1042/1 -> cfblk6/1(emi_1607)
  cfblk6/1(emi_1608) -> cyemi_1044/1
  emi_1611/1 -> cfblk6/Action
  emi_1611/2 -> emi_1609/Action
  emi_1612/1 -> emi_1611/1

== system sampleModel7293_pp_1_1_mu/cfblk198/cfblk18 ==
  cfblk1 : Inport
  cfblk14 : Inport  Port=2
  Action Port : ActionPort  ActionType=then
  cfblk10 : Delay
  cfblk11 : simulink/Discrete/Transfer Fcn Lead or Lag  PoleZ=0.95  ZeroZ=0.75  ICPrevOutput=0.0  ICPrevInput=0.0  DoSatur=off
      settings: SourceProductName=Simulink  SourceProductBaseCode=SL
  cfblk12 : Subsystem  TreatAsAtomicUnit=on
  cfblk13 : Subsystem  TreatAsAtomicUnit=on
  cfblk17 : Delay
  cfblk3 : Delay
  cfblk4 : simulink/Discrete/Difference  ICPrevInput=0.0  OutMin=[]  OutMax=[]  OutDataTypeStr=double  OutputDataTypeScalingMode=double  OutDataType=fixdt(1, 16)  OutScaling=2^-10  DoSatur=off
  cfblk5 : Subsystem  TreatAsAtomicUnit=on
  cfblk6 : DiscreteStateSpace  SampleTime=-1
  cfblk7 : Delay  DelayLengthSource=Input port
      settings: InputPortMap=u0,p1
  cfblk8 : DiscreteTransferFcn
  cfblk9 : Subsystem  TreatAsAtomicUnit=on
  cyemi_{1048..1060} (13 alike) : DataTypeConversion  OutDataTypeStr=double
  emi_1346 : Subsystem  TreatAsAtomicUnit=on
  emi_{578,1348,1461,1647} (4 alike) : If  IfExpression=Inf <= u1
  emi_{579,1349,1462,1648} (4 alike) : DataTypeConversion  OutDataTypeStr=double
  emi_1459 : Subsystem  TreatAsAtomicUnit=on
  emi_1645 : Subsystem  TreatAsAtomicUnit=on
  emi_576 : Subsystem  TreatAsAtomicUnit=on
  cfblk2 : Outport
  cfblk15 : Outport  Port=2
  cfblk16 : Outport  Port=3
  wires:
  cfblk4/1 -> cfblk16/1
  cyemi_1048/1 -> cfblk10/1
  cfblk3/1 -> cyemi_1048/1
  cyemi_1049/1 -> cfblk11/1
  cfblk10/1 -> cyemi_1049/1
  cfblk6/1 -> cyemi_1050/1
  cfblk11/1 -> cyemi_1051/1
  cyemi_1052/1 -> cfblk17/1
  cyemi_1053/1 -> cfblk3/1
  cfblk7/1 -> cyemi_1053/1, emi_1462/1
  cyemi_1054/1 -> cfblk4/1
  cfblk1/1 -> cyemi_1055/1
  cyemi_1056/1 -> cfblk6/1
  cfblk17/1 -> cyemi_1056/1
  cyemi_1057/1 -> cfblk7/1
  cfblk8/1 -> cyemi_1057/1
  cyemi_1058/1 -> cfblk7/2
  cyemi_1059/1 -> cfblk8/1
  cfblk14/1 -> cyemi_1060/1
  cyemi_1055/1 -> cfblk5/1(emi_574)
  cfblk5/1(emi_575) -> cyemi_1054/1, emi_1648/1
  emi_578/1 -> cfblk5/Action
  emi_578/2 -> emi_576/Action
  emi_579/1 -> emi_578/1
  cyemi_1051/1 -> cfblk13/1(emi_1344)
  cfblk13/1(emi_1345) -> cfblk2/1
  emi_1348/1 -> cfblk13/Action
  emi_1348/2 -> emi_1346/Action
  emi_1349/1 -> emi_1348/1
  cyemi_1050/1 -> cfblk12/1(emi_1457)
  cfblk12/1(emi_1458) -> cyemi_1052/1
  emi_1461/1 -> cfblk12/Action
  emi_1461/2 -> emi_1459/Action
  emi_1462/1 -> emi_1461/1
  cyemi_1060/1 -> cfblk9/1(emi_1643)
  cfblk9/1(emi_1644) -> emi_1349/1, emi_579/1, cyemi_1059/1, cyemi_1058/1, cfblk15/1
  emi_1647/1 -> cfblk9/Action
  emi_1647/2 -> emi_1645/Action
  emi_1648/1 -> emi_1647/1

== system sampleModel7293_pp_1_1_mu/cfblk198/cfblk19 ==
  cfblk1 : Inport
  cfblk9 : Inport  Port=2
  cfblk10 : Inport  Port=3
  Action Port : ActionPort  ActionType=else
  cfblk3 : simulink/Discrete/Difference  ICPrevInput=0.0  OutMin=[]  OutMax=[]  OutDataTypeStr=double  OutputDataTypeScalingMode=double  OutDataType=fixdt(1, 16)  OutScaling=2^-10  DoSatur=off
  cfblk4 : simulink/Continuous/PID Controller  Controller=PID  TimeDomain=Discrete-time  SampleTime=-1  IntegratorMethod=Forward Euler  FilterMethod=Forward Euler  Form=Parallel  UseFilter=on  ControllerParametersSource=internal  P=1  I=1  D=0  N=100  InitialConditionSource=internal  InitialConditionForIntegrator=0  InitialConditionForFilter=0  ExternalReset=none  LimitOutput=off  UpperSaturationLimit=inf  LowerSaturationLimit=-inf  LinearizeAsGain=off  AntiWindupMode=none  Kb=1  TrackingMode=off  Kt=1  PParamMin=[]  PParamMax=[]  IParamMin=[]  IParamMax=[]  DParamMin=[]  DParamMax=[]  NParamMin=[]  NParamMax=[]  KbParamMin=[]  KbParamMax=[]  KtParamMin=[]  KtParamMax=[]  POutMin=[]  POutMax=[]  IOutMin=[]  IOutMax=[]  DOutMin=[]  DOutMax=[]  NOutMin=[]  NOutMax=[]  KbOutMin=[]  KbOutMax=[]  KtOutMin=[]  KtOutMax=[]  IntegratorOutMin=[]  IntegratorOutMax=[]  FilterOutMin=[]  FilterOutMax=[]  SumOutMin=[]  SumOutMax=[]  SumI1OutMin=[]  SumI1OutMax=[]  SumI2OutMin=[]  SumI2OutMax=[]  SumI3OutMin=[]  SumI3OutMax=[]  SumDOutMin=[]  SumDOutMax=[]  SaturationOutMin=[]  SaturationOutMax=[]  IntegratorContinuousStateAttributes=''  IntegratorStateMustResolveToSignalObject=off  IntegratorRTWStateStorageClass=Auto  FilterContinuousStateAttributes=''  FilterStateMustResolveToSignalObject=off  FilterRTWStateStorageClass=Auto  DifferentiatorICPrevScaledInput=0  DifferentiatorOutMin=[]  DifferentiatorOutMax=[]  FilterDiffOutCoefMin=[]  FilterDiffOutCoefMax=[]  SumDenOutMin=[]  SumDenOutMax=[]  SumNumOutMin=[]  SumNumOutMax=[]  ReciprocalOutMin=[]  ReciprocalOutMax=[]  DivideOutMin=[]  DivideOutMax=[]  TunerSelectOption=Transfer Function Based (PID Tuner App)
  cfblk5 : simulink/Discrete/Transfer Fcn First Order  PoleZ=0.95  ICPrevOutput=0.0  DoSatur=off
      settings: SourceProductName=Simulink
  cfblk6 : simulink/Discrete/Transfer Fcn First Order  PoleZ=0.95  ICPrevOutput=0.0  DoSatur=off
      settings: SourceProductName=Simulink
  cfblk7 : Subsystem  TreatAsAtomicUnit=on
  cfblk8 : Delay
  cyemi_{1064..1069} (6 alike) : DataTypeConversion  OutDataTypeStr=double
  emi_877 : Subsystem  TreatAsAtomicUnit=on
  emi_879 : If  IfExpression=Inf <= u1
  emi_880 : DataTypeConversion  OutDataTypeStr=double
  cfblk2 : Outport
  wires:
  cfblk6/1 -> cfblk2/1
  cyemi_1064/1 -> cfblk3/1
  cfblk9/1 -> cyemi_1064/1
  cyemi_1065/1 -> cfblk4/1
  cyemi_1066/1 -> cfblk5/1
  cfblk8/1 -> cyemi_1066/1, emi_880/1
  cyemi_1067/1 -> cfblk6/1
  cfblk5/1 -> cyemi_1067/1
  cfblk10/1 -> cyemi_1068/1
  cyemi_1069/1 -> cfblk8/1
  cfblk1/1 -> cyemi_1069/1
  cyemi_1068/1 -> cfblk7/1(emi_875)
  cfblk7/1(emi_876) -> cyemi_1065/1
  emi_879/1 -> cfblk7/Action
  emi_879/2 -> emi_877/Action
  emi_880/1 -> emi_879/1

== system sampleModel7293_pp_1_1_mu/cfblk198/cfblk20 ==
  emi_8 : Inport
  Action Port : ActionPort  ActionType=then
  cfblk20 : Delay
  emi_9 : Outport
  wires:
  emi_8/1 -> cfblk20/1
  cfblk20/1 -> emi_9/1

== system sampleModel7293_pp_1_1_mu/cfblk198/cfblk21 ==
  emi_15 : Inport
  Action Port : ActionPort  ActionType=then
  cfblk21 : Delay
  emi_16 : Outport
  wires:
  emi_15/1 -> cfblk21/1
  cfblk21/1 -> emi_16/1

== system sampleModel7293_pp_1_1_mu/cfblk198/cfblk23 ==
  emi_1550 : Inport
  Action Port : ActionPort  ActionType=then
  cfblk23 : Delay
  emi_1551 : Outport
  wires:
  emi_1550/1 -> cfblk23/1
  cfblk23/1 -> emi_1551/1

== system sampleModel7293_pp_1_1_mu/cfblk198/cfblk24 ==
  emi_1135 : Inport
  Action Port : ActionPort  ActionType=then
  cfblk24 : Delay
  emi_1136 : Outport
  wires:
  emi_1135/1 -> cfblk24/1
  cfblk24/1 -> emi_1136/1

== system sampleModel7293_pp_1_1_mu/cfblk198/cfblk27 ==
  emi_632 : Inport
  Action Port : ActionPort  ActionType=then
  cfblk27 : Delay
  emi_633 : Outport
  wires:
  emi_632/1 -> cfblk27/1
  cfblk27/1 -> emi_633/1

== system sampleModel7293_pp_1_1_mu/cfblk198/cfblk28 ==
  emi_1029 : Inport
  Action Port : ActionPort  ActionType=then
  cfblk28 : Delay
  emi_1030 : Outport
  wires:
  emi_1029/1 -> cfblk28/1
  cfblk28/1 -> emi_1030/1

== system sampleModel7293_pp_1_1_mu/cfblk198/cfblk29 ==
  emi_681 : Inport
  Action Port : ActionPort  ActionType=then
  cfblk29 : Delay
  emi_682 : Outport
  wires:
  emi_681/1 -> cfblk29/1
  cfblk29/1 -> emi_682/1

== system sampleModel7293_pp_1_1_mu/cfblk198/cfblk6 ==
  emi_1493 : Inport
  Action Port : ActionPort  ActionType=then
  cfblk6 : simulink/Discrete/Transfer Fcn First Order  PoleZ=0.95  ICPrevOutput=0.0  DoSatur=off
      settings: SourceProductName=Simulink
  emi_1494 : Outport
  wires:
  emi_1493/1 -> cfblk6/1
  cfblk6/1 -> emi_1494/1

== system sampleModel7293_pp_1_1_mu/cfblk198/cfblk8 ==
  emi_846 : Inport
  Action Port : ActionPort  ActionType=then
  cfblk8 : simulink/Discrete/Transfer Fcn Lead or Lag  PoleZ=0.95  ZeroZ=0.75  ICPrevOutput=0.0  ICPrevInput=0.0  DoSatur=off
      settings: SourceProductName=Simulink  SourceProductBaseCode=SL
  emi_847 : Outport
  wires:
  emi_846/1 -> cfblk8/1
  cfblk8/1 -> emi_847/1

== system sampleModel7293_pp_1_1_mu/cfblk198/emi_10 ==
  Action Port : ActionPort  ActionType=else
  emi_11 : Assertion

== system sampleModel7293_pp_1_1_mu/cfblk198/emi_1031 ==
  Action Port : ActionPort  ActionType=else
  emi_1032 : Assertion

== system sampleModel7293_pp_1_1_mu/cfblk198/emi_1137 ==
  Action Port : ActionPort  ActionType=else
  emi_1138 : Assertion

== system sampleModel7293_pp_1_1_mu/cfblk198/emi_1495 ==
  Action Port : ActionPort  ActionType=else
  emi_1496 : Assertion

== system sampleModel7293_pp_1_1_mu/cfblk198/emi_1552 ==
  Action Port : ActionPort  ActionType=else
  emi_1553 : Assertion

== system sampleModel7293_pp_1_1_mu/cfblk198/emi_17 ==
  Action Port : ActionPort  ActionType=else
  emi_18 : Assertion

== system sampleModel7293_pp_1_1_mu/cfblk198/emi_634 ==
  Action Port : ActionPort  ActionType=else
  emi_635 : Assertion

== system sampleModel7293_pp_1_1_mu/cfblk198/emi_683 ==
  Action Port : ActionPort  ActionType=else
  emi_684 : Assertion

== system sampleModel7293_pp_1_1_mu/cfblk198/emi_848 ==
  Action Port : ActionPort  ActionType=else
  emi_849 : Assertion

== system sampleModel7293_pp_1_1_mu/cfblk199/cfblk12 ==
  cfblk1 : Inport
  Action Port : ActionPort  ActionType=then
  cfblk11 : Delay
  cfblk3 : simulink/Discrete/Transfer Fcn Lead or Lag  PoleZ=0.95  ZeroZ=0.75  ICPrevOutput=0.0  ICPrevInput=0.0  DoSatur=off
      settings: SourceProductName=Simulink  SourceProductBaseCode=SL
  cfblk4 : simulink/Continuous/PID Controller (2DOF)  Controller=PID  TimeDomain=Discrete-time  SampleTime=-1  IntegratorMethod=Forward Euler  FilterMethod=Forward Euler  Form=Parallel  UseFilter=on  ControllerParametersSource=internal  P=1  I=1  D=0  N=100  b=1  c=1  InitialConditionSource=internal  InitialConditionForIntegrator=0  InitialConditionForFilter=0  ExternalReset=none  LimitOutput=off  UpperSaturationLimit=inf  LowerSaturationLimit=-inf  LinearizeAsGain=off  AntiWindupMode=none  Kb=1  TrackingMode=off  Kt=1  PParamMin=[]  PParamMax=[]  IParamMin=[]  IParamMax=[]  DParamMin=[]  DParamMax=[]  NParamMin=[]  NParamMax=[]  bParamMin=[]  bParamMax=[]  cParamMin=[]  cParamMax=[]  KbParamMin=[]  KbParamMax=[]  KtParamMin=[]  KtParamMax=[]  POutMin=[]  POutMax=[]  IOutMin=[]  IOutMax=[]  DOutMin=[]  DOutMax=[]  NOutMin=[]  NOutMax=[]  bOutMin=[]  bOutMax=[]  cOutMin=[]  cOutMax=[]  KbOutMin=[]  KbOutMax=[]  KtOutMin=[]  KtOutMax=[]  IntegratorOutMin=[]  IntegratorOutMax=[]  FilterOutMin=[]  FilterOutMax=[]  SumOutMin=[]  SumOutMax=[]  Sum1OutMin=[]  Sum1OutMax=[]  Sum2OutMin=[]  Sum2OutMax=[]  Sum3OutMin=[]  Sum3OutMax=[]  SumI1OutMin=[]  SumI1OutMax=[]  SumI2OutMin=[]  SumI2OutMax=[]  SumI3OutMin=[]  SumI3OutMax=[]  SumDOutMin=[]  SumDOutMax=[]  SaturationOutMin=[]  SaturationOutMax=[]  IntegratorContinuousStateAttributes=''  IntegratorStateMustResolveToSignalObject=off  IntegratorRTWStateStorageClass=Auto  FilterContinuousStateAttributes=''  FilterStateMustResolveToSignalObject=off  FilterRTWStateStorageClass=Auto  DifferentiatorICPrevScaledInput=0  DifferentiatorOutMin=[]  DifferentiatorOutMax=[]  FilterDiffOutCoefMin=[]  FilterDiffOutCoefMax=[]  SumDenOutMin=[]  SumDenOutMax=[]  SumNumOutMin=[]  SumNumOutMax=[]  ReciprocalOutMin=[]  ReciprocalOutMax=[]  DivideOutMin=[]  DivideOutMax=[]  TunerSelectOption=Transfer Function Based (PID Tuner App)
  cfblk5 : Subsystem  TreatAsAtomicUnit=on
  cfblk6 : Delay  ShowEnablePort=on
      settings: InputPortMap=u0,e6
  cfblk7 : Subsystem  TreatAsAtomicUnit=on
  cfblk8 : DiscreteIntegrator  SampleTime=-1  OutDataTypeStr=double  ICPrevOutput=DiscIntNeverNeededParam  ICPrevScaledInput=DiscIntNeverNeededParam
  cyemi_{1093..1101} (9 alike) : DataTypeConversion  OutDataTypeStr=double
  emi_1681 : Subsystem  TreatAsAtomicUnit=on
  emi_1683 : If  IfExpression=Inf <= u1
  emi_1684 : DataTypeConversion  OutDataTypeStr=double
  emi_734 : Subsystem  TreatAsAtomicUnit=on
  emi_736 : If  IfExpression=Inf <= u1
  emi_737 : DataTypeConversion  OutDataTypeStr=double
  cfblk2 : Outport
  cfblk9 : Outport  Port=2
  cfblk10 : Outport  Port=3
  wires:
  cfblk8/1 -> cfblk2/1
  cfblk4/1 -> cfblk9/1, cfblk10/1, cyemi_1099/1
  cyemi_1093/1 -> cfblk11/1
  cyemi_1094/1 -> cfblk3/1
  cfblk1/1 -> cyemi_1094/1
  cyemi_1095/1 -> cfblk4/1
  cyemi_1096/1 -> cfblk4/2
  cfblk6/1 -> cyemi_1097/1, emi_737/1
  cyemi_1098/1 -> cfblk6/1
  cfblk11/1 -> cyemi_1098/1
  cyemi_1099/1 -> cfblk6/2
  cfblk3/1 -> cyemi_1100/1
  cyemi_1101/1 -> cfblk8/1
  cyemi_1097/1 -> cfblk5/1(emi_732)
  cfblk5/1(emi_733) -> cyemi_1093/1, emi_1684/1
  emi_736/1 -> cfblk5/Action
  emi_736/2 -> emi_734/Action
  emi_737/1 -> emi_736/1
  cyemi_1100/1 -> cfblk7/1(emi_1679)
  cfblk7/1(emi_1680) -> cyemi_1101/1, cyemi_1096/1, cyemi_1095/1
  emi_1683/1 -> cfblk7/Action
  emi_1683/2 -> emi_1681/Action
  emi_1684/1 -> emi_1683/1
